simulink model "Target_Control_System"  (R2021b)
settings: Solver=FixedStepDiscrete  StartTime=0.0  StopTime=5  RelTol=1e-3
PreLoadFcn:
  | RTWConfigurationCB('preloadfcn', bdroot);
PostLoadFcn:
  | load('configuration/data_struct.mat');
  | load('configuration/fluxMaps_propMotor.mat');
  | load('configuration/parameterInit_PROP.mat');
  | load('configuration/parameterInit_PUMP.mat');
  | load('configuration/parameterInit_PITCH.mat');
  | load('configuration/parameterInit_TILT.mat');
  | %load('configuration/base_workspace_signal_definition.mat');
  | %load('resolvedatastores_to_baseworkspace_for_faster_simulation.mat');
model workspace (MAT data in the model file):
  SIMULATION_OPTIONS : Simulink.Parameter (value not decoded)
  TARGET_CODE_GEN : Simulink.Parameter (value not decoded)
  TCS_SAMPLE_FREQ_HZ : Simulink.Parameter (value not decoded)
symbols that are objects in the model workspace (value not decoded): TARGET_CODE_GEN, TCS_SAMPLE_FREQ_HZ
undefined symbols (not defined in the file): A_DQ_REF_LPF_INIT__PITCH, A_DQ_REF_LPF_INIT__PROP, A_DQ_REF_LPF_INIT__PUMP, A_DQ_REF_LPF_INIT__TILT, A_OBSERVER_CONFIDENCE_INIT__PITCH, A_OBSERVER_CONFIDENCE_INIT__PROP, A_OBSERVER_CONFIDENCE_INIT__PUMP, A_OBSERVER_CONFIDENCE_INIT__TILT, ACTUATOR_MAX_ANGLE_TRIP__PITCH, ACTUATOR_MIN_ANGLE_TRIP__PITCH, ACTUATOR_POS_SENSOR_INV_DIRECTION__PITCH, ACTUATOR_POS_SENSOR_INV_DIRECTION__TILT, ACTUATOR_POS_SENSOR_OFFSET__PITCH, ACTUATOR_POS_SENSOR_OFFSET__TILT, ADC_scaler1_baseaddr_TILT, ADC_SCALER_FLOAT_TO_FIXPOINT_EXPANSION, ANGLE_ELEC_FROM_SENSOR_OFFSET_INIT__PITCH, ANGLE_ELEC_FROM_SENSOR_OFFSET_INIT__PROP, ANGLE_ELEC_FROM_SENSOR_OFFSET_INIT__PUMP, ANGLE_ELEC_FROM_SENSOR_OFFSET_INIT__TILT, AUTO_CLEAR_FAULTS_ENABLED__PITCH, AUTO_CLEAR_FAULTS_ENABLED__PROP, AUTO_CLEAR_FAULTS_ENABLED__PUMP, AUTO_CLEAR_FAULTS_ENABLED__TILT, AUTO_CLEAR_FAULTS_WAIT_TICKS__PITCH, AUTO_CLEAR_FAULTS_WAIT_TICKS__PROP, AUTO_CLEAR_FAULTS_WAIT_TICKS__PUMP, AUTO_CLEAR_FAULTS_WAIT_TICKS__TILT, AUTO_I_ZERO_IDLE_TICKS__PITCH, AUTO_I_ZERO_IDLE_TICKS__PROP, AUTO_I_ZERO_IDLE_TICKS__PUMP, AUTO_I_ZERO_IDLE_TICKS__TILT, AUTO_I_ZERO_OFFSET_IDC_THRESHOLD__PITCH, AUTO_I_ZERO_OFFSET_IDC_THRESHOLD__PROP, AUTO_I_ZERO_OFFSET_IDC_THRESHOLD__PUMP, AUTO_I_ZERO_OFFSET_IDC_THRESHOLD__TILT, AUTO_I_ZERO_OFFSET_IPH_THRESHOLD__PITCH, AUTO_I_ZERO_OFFSET_IPH_THRESHOLD__PROP, AUTO_I_ZERO_OFFSET_IPH_THRESHOLD__PUMP, AUTO_I_ZERO_OFFSET_IPH_THRESHOLD__TILT, AUTO_SENSORLESS_SWITCHOVER_DISABLE_OMEGA, AUTO_SENSORLESS_SWITCHOVER_ENABLE_OMEGA, AUTO_SENSORLESS_SWITCHOVER_MIN_CONFIDENCE, AUXILIARY_PROTECTION_UNIT_BASEADDR__TILT, blanking_max_error_omega_INIT_PITCH, blanking_max_error_omega_INIT_TILT, blanking_max_error_position_INIT_PITCH, blanking_max_error_position_INIT_TILT, BRUTE_START_I_Q_REF_RAMP_SPEED__PITCH, BRUTE_START_I_Q_REF_RAMP_SPEED__PROP, BRUTE_START_I_Q_REF_RAMP_SPEED__PUMP, BRUTE_START_I_Q_REF_RAMP_SPEED__TILT, CONTROL_LOOP_DT_INIT__PITCH, CONTROL_LOOP_DT_INIT__PROP, CONTROL_LOOP_DT_INIT__PUMP, CONTROL_LOOP_DT_INIT__TILT, CORRECTION_FILTER_SCALE__PITCH, CORRECTION_FILTER_SCALE__PROP, CORRECTION_FILTER_SCALE__PUMP, CORRECTION_FILTER_SCALE__TILT ... (+458)
libraries: simulink x178, Reusables_Lib x24
(part 7 of 47)

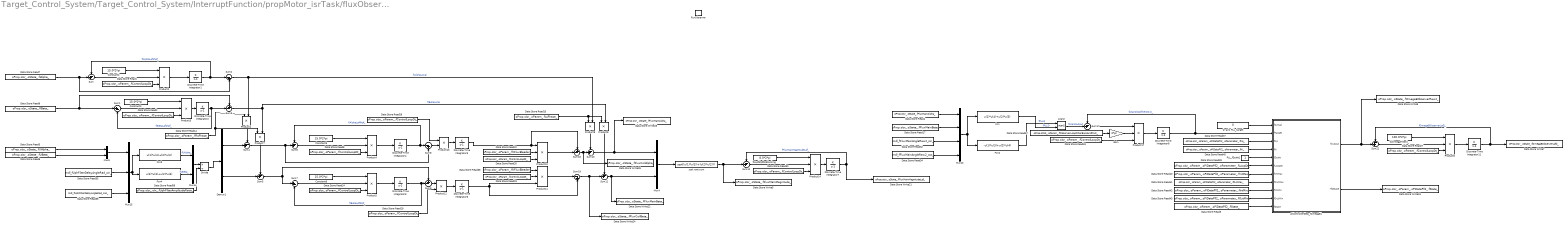
== system Target_Control_System/Target_Control_System/InterruptFunction/propMotor_isrTask/fluxObserver ==
  fluxObserver : TriggerPort  TriggerType=function-call  VariantControl=Variant
  Atan2 : Trigonometry  Operator=atan2
  Constant{2..3,5..6} (4 alike) : Constant  Value=15.0*2*pi  OutDataTypeStr=single  SampleTime=-1
  Data Store Read{1..2,8,20,23..24,27..30,33} (11 alike) : DataStoreRead  DataStoreName=oProp  DataStoreElements=oProp.oIsr_.oParam_.fControlLoopDt_  IndexOptions=Index vector (dialog)  Indices=1  OutputSizes=1
  Data Store Read14 : DataStoreRead  DataStoreName=oProp  DataStoreElements=oProp.oIsr_.oParam_.fRsPhase_  IndexOptions=Index vector (dialog)  Indices=1  OutputSizes=1
  Data Store Read15 : DataStoreRead  DataStoreName=oProp  DataStoreElements=oProp.oIsr_.oParam_.fLsPhase_  IndexOptions=Index vector (dialog)  Indices=1  OutputSizes=1
  Data Store Read17 : DataStoreRead  DataStoreName=oProp  DataStoreElements=oProp.oIsr_.oState_.fFluxMainBeta_  IndexOptions=Index vector (dialog)  Indices=1  OutputSizes=1
  Data Store Read22 : DataStoreRead  DataStoreName=oProp  DataStoreElements=oProp.oIsr_.oParam_.fKFluxBleeder_  IndexOptions=Index vector (dialog)  Indices=1  OutputSizes=1
  Data Store Read3 : DataStoreRead  DataStoreName=oProp  DataStoreElements=oProp.oIsr_.oParam_.oPiDataPll2_.fState_  IndexOptions=Index vector (dialog)  Indices=1  OutputSizes=1
  Data Store Read32 : DataStoreRead  DataStoreName=mdl_fFluxMainAngleRaw2_sin_  IndexOptions=Index vector (dialog)  Indices=1  OutputSizes=1
  Data Store Read34 : DataStoreRead  DataStoreName=mdl_fFluxMainAngleRaw2_cos_  IndexOptions=Index vector (dialog)  Indices=1  OutputSizes=1
  Data Store Read35 : DataStoreRead  DataStoreName=mdl_fUphFilterDelayAngleRad_sin_  IndexOptions=Index vector (dialog)  Indices=1  OutputSizes=1
  Data Store Read36 : DataStoreRead  DataStoreName=mdl_fUphFilterDelayAngleRad_cos_  IndexOptions=Index vector (dialog)  Indices=1  OutputSizes=1
  Data Store Read37 : DataStoreRead  DataStoreName=oProp  DataStoreElements=oProp.oIsr_.oParam_.oPiDataPll2_.oParameter_.fKp_  IndexOptions=Index vector (dialog)  Indices=1  OutputSizes=1
  Data Store Read38 : DataStoreRead  DataStoreName=oProp  DataStoreElements=oProp.oIsr_.oParam_.fKFluxBleeder_  IndexOptions=Index vector (dialog)  Indices=1  OutputSizes=1
  Data Store Read39 : DataStoreRead  DataStoreName=oProp  DataStoreElements=oProp.oIsr_.oParam_.oPiDataPll2_.oParameter_.fLoopDt_  IndexOptions=Index vector (dialog)  Indices=1  OutputSizes=1
  Data Store Read4 : DataStoreRead  DataStoreName=oProp  DataStoreElements=oProp.oIsr_.oState_.fFluxMainAlpha_  IndexOptions=Index vector (dialog)  Indices=1  OutputSizes=1
  Data Store Read40 : DataStoreRead  DataStoreName=oProp  DataStoreElements=oProp.oIsr_.oParam_.oPiDataPll2_.oParameter_.fIntMax_  IndexOptions=Index vector (dialog)  Indices=1  OutputSizes=1
  Data Store Read41 : DataStoreRead  DataStoreName=oProp  DataStoreElements=oProp.oIsr_.oParam_.oPiDataPll2_.oParameter_.fOutMax_  IndexOptions=Index vector (dialog)  Indices=1  OutputSizes=1
  Data Store Read42 : DataStoreRead  DataStoreName=oProp  DataStoreElements=oProp.oIsr_.oParam_.oPiDataPll2_.oParameter_.fIntMin_  IndexOptions=Index vector (dialog)  Indices=1  OutputSizes=1
  Data Store Read43 : DataStoreRead  DataStoreName=oProp  DataStoreElements=oProp.oIsr_.oParam_.oPiDataPll2_.oParameter_.fOutMin_  IndexOptions=Index vector (dialog)  Indices=1  OutputSizes=1
  Data Store Read45 : DataStoreRead  DataStoreName=oProp  DataStoreElements=oProp.oIsr_.oParam_.oPiDataPll2_.oParameter_.fKi_  IndexOptions=Index vector (dialog)  Indices=1  OutputSizes=1
  Data Store Read5 : DataStoreRead  DataStoreName=oProp  DataStoreElements=oProp.oIsr_.oState_.fUAlpha_  IndexOptions=Index vector (dialog)  Indices=1  OutputSizes=1
  Data Store Read57 : DataStoreRead  DataStoreName=oProp  DataStoreElements=oProp.oMot_.oParam_.fObserverLoopFilterBandwidthHz_  IndexOptions=Index vector (dialog)  Indices=1  OutputSizes=1
  Data Store Read58 : DataStoreRead  DataStoreName=oProp  DataStoreElements=oProp.oIsr_.oIn_.fUphFilterAmplitudeRatio_  IndexOptions=Index vector (dialog)  Indices=1  OutputSizes=1
  Data Store Read6 : DataStoreRead  DataStoreName=oProp  DataStoreElements=oProp.oIsr_.oState_.fUBeta_  IndexOptions=Index vector (dialog)  Indices=1  OutputSizes=1
  Data Store Read7 : DataStoreRead  DataStoreName=oProp  DataStoreElements=oProp.oIsr_.oState_.fIAlpha_  IndexOptions=Index vector (dialog)  Indices=1  OutputSizes=1
  Data Store Read9 : DataStoreRead  DataStoreName=oProp  DataStoreElements=oProp.oIsr_.oState_.fIBeta_  IndexOptions=Index vector (dialog)  Indices=1  OutputSizes=1
  Data Store Write19 : DataStoreWrite  DataStoreName=oProp  DataStoreElements=oProp.oIsr_.oParam_.oPiDataPll2_.fState_  IndexOptions=Index vector (dialog)  Indices=1  OutputSizes=1
  Data Store Write21 : DataStoreWrite  DataStoreName=oProp  DataStoreElements=oProp.oIsr_.oState_.fFluxMainMagnitudeLpf_  IndexOptions=Index vector (dialog)  Indices=1  OutputSizes=1
  Data Store Write22 : DataStoreWrite  DataStoreName=oProp  DataStoreElements=oProp.oIsr_.oState_.fFluxMainBeta_  IndexOptions=Index vector (dialog)  Indices=1  OutputSizes=1
  Data Store Write23 : DataStoreWrite  DataStoreName=oProp  DataStoreElements=oProp.oIsr_.oState_.fFluxMainAlpha_  IndexOptions=Index vector (dialog)  Indices=1  OutputSizes=1
  Data Store Write24 : DataStoreWrite  DataStoreName=oProp  DataStoreElements=oProp.oIsr_.oState_.fFluxCoilBeta_  IndexOptions=Index vector (dialog)  Indices=1  OutputSizes=1
  Data Store Write26 : DataStoreWrite  DataStoreName=oProp  DataStoreElements=oProp.oIsr_.oState_.fFluxCoilAlpha_  IndexOptions=Index vector (dialog)  Indices=1  OutputSizes=1
  Data Store Write5 : DataStoreWrite  DataStoreName=oProp  DataStoreElements=oProp.oIsr_.oState_.fFluxMainMagnitude_  IndexOptions=Index vector (dialog)  Indices=1  OutputSizes=1
  Data Store Write7 : DataStoreWrite  DataStoreName=oProp  DataStoreElements=oProp.oIsr_.oState_.fOmegaEObserverLpf2_  IndexOptions=Index vector (dialog)  Indices=1  OutputSizes=1
  Data Store Write9 : DataStoreWrite  DataStoreName=oProp  DataStoreElements=oProp.oIsr_.oState_.fOmegaEObserverRaw2_  IndexOptions=Index vector (dialog)  Indices=1  OutputSizes=1
  Demux1 : Demux  Outputs=2
  Discrete-Time Integrator{1..2,4..9,11} (9 alike) : DiscreteIntegrator  IntegratorMethod=Accumulation: Forward Euler  SampleTime=-1  OutDataTypeStr=single  UpperSaturationLimit=2*pi*100  LowerSaturationLimit=-2*pi*100  ICPrevOutput=DiscIntNeverNeededParam  ICPrevScaledInput=DiscIntNeverNeededParam
  Divide : Product  Inputs=*/
  Fcn : Fcn  Expr=u(1)*u(4)+u(2)*u(3)
  Fcn2 : Fcn  Expr=-u(1)*u(3)+u(2)*u(4)
  Fcn3 : Fcn  Expr=u(1)*u(4)-u(2)*u(3)
  Fcn4 : Fcn  Expr=u(1)*u(3)+u(2)*u(4)
  Gain : Gain  Gain=2*pi
  Mux13 : Mux
  Mux14 : Mux  Inputs=2
  Mux15 : Mux  Inputs=3
  Mux4 : Mux  Inputs=2
  Mux5 : Mux  Inputs=2
  PLL_fScale1 : Constant  OutDataTypeStr=single  SampleTime=-1
  Product{1,7..9,12..13} (6 alike) : Product
  Product{2..6,10..11,14,17} (9 alike) : Product  Inputs=3
  Q-axis PLL_target : Constant  Value=0  OutDataTypeStr=single  SampleTime=-1
  Sum{,4..6,10..12,17,22} (9 alike) : Sum  Inputs=-+|
  Sum1 : Sum  Inputs=|+-
  Sum18 : Sum  Inputs=+-|
  Sum19 : Sum  Inputs=|-+
  Sum2 : Sum  Inputs=|-+
  Sum3 : Sum  Inputs=+-|
  Sum7 : Sum  Inputs=|+-
  Sum8 : Sum  Inputs=|-+
  Sum9 : Sum  Inputs=+-|
  fALpf4hpfDcBlocking : Constant  Value=8.0*2*pi  OutDataTypeStr=single  SampleTime=-1
  fAOmegaFilter2_ : Constant  Value=100.0*2*pi  OutDataTypeStr=single  SampleTime=-1
  piControllerStep_fOmegaE1 : Subsystem
  sqrt root sum : Fcn  Expr=sqrt((u(1)*u(1))+(u(2)*u(2)))
  wires:
  Data Store Read29/1 -> Product12/2
  Data Store Read35/1 -> Mux15/2
  Data Store Read24/1 -> Product5/3
  Constant5/1 -> Product4/1
  Mux15/1 -> Fcn4/1, Fcn3/1
  Product7/1 -> Sum5/1
  Data Store Read57/1 -> Gain/1
  Mux4/1 -> sqrt root sum/1
  Discrete-Time Integrator2/1 -> Sum1/2, Sum3/2  "fIBetaLpf4hpf_"
  Constant6/1 -> Product5/1
  Sum3/1 -> Product9/2, Product7/2  "fIBetaLocal"
  Sum7/1 -> Product5/2
  Sum2/1 -> Product1/2, Product8/2  "fIAlphaLocal"
  Data Store Read5/1 -> Mux5/1
  Product11/1 -> Sum19/1
  Sum6/1 -> Product4/2
  Discrete-Time Integrator1/1 -> Sum2/1, Sum/1  "fIAlphaLpf4hpf_"
  fALpf4hpfDcBlocking/1 -> Product14/1
  Sum10/1 -> Mux4/1, Data Store Write23/1
  Data Store Read28/1 -> Product13/1
  Sum1/1 -> Product3/2
  Data Store Read1/1 -> Product2/3
  Data Store Read43/1 -> piControllerStep_fOmegaE1/10(fOutMin)
  Demux1/1 -> Sum4/2
  Data Store Read38/1 -> Product11/1
  Discrete-Time Integrator6/1 -> Sum19/2, Product11/3
  Divide/1 -> Demux1/1
  Product13/1 -> Discrete-Time Integrator5/1
  Data Store Read36/1 -> Mux15/3
  Mux14/1 -> Divide/1
  Data Store Read40/1 -> piControllerStep_fOmegaE1/7(fIntMax)
  Data Store Read45/1 -> piControllerStep_fOmegaE1/4(fKi)
  fAOmegaFilter2_/1 -> Product6/1
  Data Store Read17/1 -> Mux13/2
  Product1/1 -> Sum4/1
  Data Store Read39/1 -> piControllerStep_fOmegaE1/6(fLoopDt)
  Data Store Read7/1 -> Sum2/2, Sum/2
  Sum19/1 -> Sum11/2, Data Store Write24/1
  Sum18/1 -> Sum10/2, Data Store Write26/1
  Data Store Read34/1 -> Mux13/4
  Product17/1 -> Discrete-Time Integrator8/1
  piControllerStep_fOmegaE1/1(fOutput) -> Sum22/2, Data Store Write9/1
  Data Store Read8/1 -> Product4/3
  Atan2/1 -> Sum17/2  "fAtan2output"
  Product2/1 -> Discrete-Time Integrator1/1
  Data Store Read14/1 -> Product1/1, Product7/1
  Fcn4/1 -> Mux14/2  "fUBeta_"
  Data Store Read20/1 -> Product10/3
  Discrete-Time Integrator5/1 -> Sum18/1, Product10/1
  Demux1/2 -> Sum5/2
  Product10/1 -> Sum18/2
  Sum17/1 -> Product17/1
  Product8/1 -> Sum10/1
  Discrete-Time Integrator11/1 -> Sum22/1, Data Store Write7/1  "fOmegaEObserverLpf2_"
  Mux13/1 -> Fcn2/1, Fcn/1
  Q-axis PLL_target/1 -> piControllerStep_fOmegaE1/1(fActual)
  Fcn3/1 -> Mux14/1  "fUAlpha_"
  Data Store Read42/1 -> piControllerStep_fOmegaE1/9(fIntMin)
  Sum4/1 -> Sum8/2, Sum6/2
  Constant3/1 -> Product3/1
  Fcn/1 -> Atan2/2  "fPLLD"
  Product6/1 -> Discrete-Time Integrator11/1
  Data Store Read2/1 -> Product3/3
  Discrete-Time Integrator9/1 -> Sum9/2, Sum7/2  "fIBetaLpf4hpf_"
  Sum5/1 -> Sum9/1, Sum7/1
  Mux5/1 -> Mux15/1
  Data Store Read58/1 -> Divide/2
  Sum12/1 -> Product14/2
  Sum22/1 -> Product6/2
  Fcn2/1 -> Atan2/1  "fPLLQ"
  sqrt root sum/1 -> Data Store Write5/1, Sum12/2
  Data Store Read23/1 -> Product11/2
  PLL_fScale1/1 -> piControllerStep_fOmegaE1/5(fScale)
  Data Store Read22/1 -> Product10/2
  Product12/1 -> Discrete-Time Integrator6/1
  Discrete-Time Integrator8/1 -> piControllerStep_fOmegaE1/2(fTarget), Sum17/1  "fAtan2loopfilter2Out_"
  Sum/1 -> Product2/2
  Sum9/1 -> Product12/1
  Data Store Read3/1 -> piControllerStep_fOmegaE1/11(fState)
  Gain/1 -> Product17/2
  Sum8/1 -> Product13/2
  Sum11/1 -> Mux4/2, Data Store Write22/1
  Data Store Read15/1 -> Product8/1, Product9/1
  Product5/1 -> Discrete-Time Integrator9/1
  Discrete-Time Integrator4/1 -> Sum8/1, Sum6/1  "fIAlphaLpf4hpf_"
  Constant2/1 -> Product2/1
  Discrete-Time Integrator7/1 -> Data Store Write21/1, Sum12/1  "fFluxMainMagnitudeLpf_"
  Data Store Read6/1 -> Mux5/2
  Data Store Read32/1 -> Mux13/3
  Data Store Read27/1 -> Product6/3
  Product4/1 -> Discrete-Time Integrator4/1
  Data Store Read4/1 -> Mux13/1
  Data Store Read33/1 -> Product17/3
  Data Store Read30/1 -> Product14/3
  piControllerStep_fOmegaE1/2(*fpState) -> Data Store Write19/1
  Data Store Read37/1 -> piControllerStep_fOmegaE1/3(fKp)
  Product9/1 -> Sum11/1
  Product3/1 -> Discrete-Time Integrator2/1
  Product14/1 -> Discrete-Time Integrator7/1
  Data Store Read41/1 -> piControllerStep_fOmegaE1/8(fOutMax)
  Data Store Read9/1 -> Sum1/1, Sum3/1

== system Target_Control_System/Target_Control_System/InterruptFunction/propMotor_isrTask/isrStateMachine ==
  isrStateMachine : TriggerPort  TriggerType=function-call  VariantControl=Variant
  ISR State Machine : Stateflow chart  TreatAsAtomicUnit=on

== system Target_Control_System/Target_Control_System/InterruptFunction/propMotor_isrTask/pwmGeneration ==
  pwmGeneration : TriggerPort  TriggerType=function-call  VariantControl=Variant
  Data Store Read9 : DataStoreRead  DataStoreName=oProp  DataStoreElements=oProp.oIsr_.oIn_.uiCurrentControllerActive_  IndexOptions=Index vector (dialog)  Indices=1  OutputSizes=1
  Subsystem : Subsystem
  wires:
  Data Store Read9/1 -> Subsystem/Enable

== system Target_Control_System/Target_Control_System/InterruptFunction/propMotor_isrTask/resetFlags ==
  resetFlags : TriggerPort  TriggerType=function-call  VariantControl=Variant
  Constant : Constant  Value=0  OutDataTypeStr=int32  SampleTime=-1
  Data Store Write1 : DataStoreWrite  DataStoreName=oProp  DataStoreElements=oProp.oIsr_.oOut_.iIBiasUpdated_  IndexOptions=Index vector (dialog)  Indices=1  OutputSizes=1
  Data Store Write12 : DataStoreWrite  DataStoreName=oProp  DataStoreElements=oProp.oIsr_.oState_.iPwmUpdated_  IndexOptions=Index vector (dialog)  Indices=1  OutputSizes=1
  Data Store Write2 : DataStoreWrite  DataStoreName=oProp  DataStoreElements=oProp.oIsr_.oOut_.iUBiasUpdated_  IndexOptions=Index vector (dialog)  Indices=1  OutputSizes=1
  wires:
  Constant/1 -> Data Store Write12/1, Data Store Write1/1, Data Store Write2/1

== system Target_Control_System/Target_Control_System/InterruptFunction/propMotor_isrTask/softCurrentLimiting ==
  softCurrentLimiting : TriggerPort  TriggerType=function-call  VariantControl=Variant
  Abs : Abs
  Abs1 : Abs
  Abs2 : Abs
  Add : Sum  Inputs=+-
  Add1 : Sum  Inputs=+-
  Add2 : Sum  Inputs=+-
  Constant : Constant  Value=0  OutDataTypeStr=single  SampleTime=-1
  Data Store Read1 : DataStoreRead  DataStoreName=oProp  DataStoreElements=oProp.oIsr_.oIn_.oAdcData_.fIa_  IndexOptions=Index vector (dialog)  Indices=1  OutputSizes=1
  Data Store Read2 : DataStoreRead  DataStoreName=oProp  DataStoreElements=oProp.oIsr_.oParam_.fSoftILimitA_  IndexOptions=Index vector (dialog)  Indices=1  OutputSizes=1
  Data Store Read3 : DataStoreRead  DataStoreName=oProp  DataStoreElements=oProp.oIsr_.oIn_.oAdcData_.fIb_  IndexOptions=Index vector (dialog)  Indices=1  OutputSizes=1
  Data Store Read4 : DataStoreRead  DataStoreName=oProp  DataStoreElements=oProp.oIsr_.oParam_.fSoftILimitA_  IndexOptions=Index vector (dialog)  Indices=1  OutputSizes=1
  Data Store Read5 : DataStoreRead  DataStoreName=oProp  DataStoreElements=oProp.oIsr_.oIn_.oAdcData_.fIc_  IndexOptions=Index vector (dialog)  Indices=1  OutputSizes=1
  Data Store Read6 : DataStoreRead  DataStoreName=oProp  DataStoreElements=oProp.oIsr_.oParam_.fSoftILimitA_  IndexOptions=Index vector (dialog)  Indices=1  OutputSizes=1
  Equal : RelationalOperator  Operator=>  OutDataTypeStr=boolean  RndMeth=Simplest
  Equal1 : RelationalOperator  Operator=>  OutDataTypeStr=boolean  RndMeth=Simplest
  Equal2 : RelationalOperator  Operator=>  OutDataTypeStr=boolean  RndMeth=Simplest
  Subsystem : Subsystem
  Switch : Switch  Criteria=u2 > Threshold
  Switch1 : Switch  Criteria=u2 > Threshold
  wires:
  Equal/1 -> Switch/2
  Data Store Read6/1 -> Add2/2
  Data Store Read5/1 -> Abs2/1
  Equal1/1 -> Switch1/2
  Abs1/1 -> Add1/1
  Add/1 -> Equal/2, Switch/3  "fMaxOvershoot"
  Constant/1 -> Equal2/2
  Abs/1 -> Add/1
  Add2/1 -> Switch1/1, Equal1/1  "fTemp"
  Switch1/1 -> Equal2/1, Subsystem/1(fMaxOvershoot)  "fMaxOvershoot"
  Data Store Read3/1 -> Abs1/1
  Add1/1 -> Switch/1, Equal/1  "fTemp"
  Switch/1 -> Switch1/3, Equal1/2  "fMaxOvershoot"
  Equal2/1 -> Subsystem/Enable
  Data Store Read1/1 -> Abs/1
  Abs2/1 -> Add2/1
  Data Store Read4/1 -> Add1/2
  Data Store Read2/1 -> Add/2

== system Target_Control_System/Target_Control_System/InterruptFunction/propMotor_setPwm/ModelSourceFPGAProp ==
  note: 1) Add Subsystem or Model blocks as valid variant choices.
      | 2) You cannot connect blocks at this level. At simulation, connectivity is automatically
      | determined, based on the active variant and port name matching.
  DoNotIncludeCustomCode : Subsystem  TreatAsAtomicUnit=on  VariantControl=TARGET_CODE_GEN == 0
  IncludeCustomCode : Subsystem  TreatAsAtomicUnit=on  VariantControl=(default)

== system Target_Control_System/Target_Control_System/InterruptFunction/propMotor_setPwm/Subsystem ==
  note: // signal to the pwm block that we handled the interrupt
  Enable : EnablePort
  Constant10 : Constant  OutDataTypeStr=int32  SampleTime=-1
  Data Store Read2 : DataStoreRead  DataStoreName=oProp  DataStoreElements=oProp.oIsr_.oParam_.fPwmPeriodTicksFloat_  IndexOptions=Index vector (dialog)  Indices=1  OutputSizes=1
  Data Store Write : DataStoreWrite  DataStoreName=oProp  DataStoreElements=oProp.oIsr_.oOut_.uiPwmDutyTicksA_  IndexOptions=Index vector (dialog)  Indices=1  OutputSizes=1
  Data Type Conversion : DataTypeConversion  OutDataTypeStr=uint32
  Shift Arithmetic1 : ArithShift  BitShiftNumberSource=Input port  BitShiftNumber=8  BitShiftDirection=Right
      settings: InputPortMap=u0,p1
  wires:
  Shift Arithmetic1/1 -> Data Type Conversion/1
  Data Type Conversion/1 -> Data Store Write/1
  Data Store Read2/1 -> Shift Arithmetic1/1
  Constant10/1 -> Shift Arithmetic1/2

== system Target_Control_System/Target_Control_System/InterruptFunction/pumpMotor_isrSchedule/Triggered Subsystem ==
  Trigger : TriggerPort  VariantControl=Variant
  Function-Call Generator : simulink/Ports & Subsystems/Function-Call Generator  sample_time=-1  numberOfIterations=1  DisallowWideOutput=off
  Output : Outport
  wires:
  Function-Call Generator/1 -> Output/1

== system Target_Control_System/Target_Control_System/InterruptFunction/pumpMotor_isrTask/abcToAlphaBeta ==
  abcToAlphaBeta : TriggerPort  TriggerType=function-call  VariantControl=Variant
  Constant1 : Constant  Value=TARGET_CODE_GEN  SampleTime=-1
  Data Store Read1 : DataStoreRead  DataStoreName=oPump  DataStoreElements=oPump.oIsr_.oState_.fUaPostlpf_  IndexOptions=Index vector (dialog)  Indices=1  OutputSizes=1
  Data Store Read13 : DataStoreRead  DataStoreName=oPump  DataStoreElements=oPump.oIsr_.oState_.fUbPostlpf_  IndexOptions=Index vector (dialog)  Indices=1  OutputSizes=1
  Data Store Read14 : DataStoreRead  DataStoreName=oPump  DataStoreElements=oPump.oIsr_.oState_.fUcPostlpf_  IndexOptions=Index vector (dialog)  Indices=1  OutputSizes=1
  Data Store Read15 : DataStoreRead  DataStoreName=oPump  DataStoreElements=oPump.oIsr_.oIn_.fUphFilterDelayAngleRad_  IndexOptions=Index vector (dialog)  Indices=1  OutputSizes=1
  Data Store Read16 : DataStoreRead  DataStoreName=oPump  DataStoreElements=oPump.oIsr_.oIn_.oAdcData_.fIa_  IndexOptions=Index vector (dialog)  Indices=1  OutputSizes=1
  Data Store Read17 : DataStoreRead  DataStoreName=oPump  DataStoreElements=oPump.oIsr_.oState_.fOmegaEObserverRaw2_  IndexOptions=Index vector (dialog)  Indices=1  OutputSizes=1
  Data Store Read19 : DataStoreRead  DataStoreName=oPump  DataStoreElements=oPump.oIsr_.oParam_.iInverseDirection_  IndexOptions=Index vector (dialog)  Indices=1  OutputSizes=1
  Data Store Read2 : DataStoreRead  DataStoreName=oPump  DataStoreElements=oPump.oIsr_.oIn_.oAdcData_.fIb_  IndexOptions=Index vector (dialog)  Indices=1  OutputSizes=1
  Data Store Read4 : DataStoreRead  DataStoreName=oPump  DataStoreElements=oPump.oIsr_.oIn_.oAdcData_.fIc_  IndexOptions=Index vector (dialog)  Indices=1  OutputSizes=1
  Data Store Read8 : DataStoreRead  DataStoreName=oPump  DataStoreElements=oPump.oIsr_.oParam_.iInverseDirection_  IndexOptions=Index vector (dialog)  Indices=1  OutputSizes=1
  Data Store Write1 : DataStoreWrite  DataStoreName=oPump  DataStoreElements=oPump.oIsr_.oState_.fIAlpha_  IndexOptions=Index vector (dialog)  Indices=1  OutputSizes=1
  Data Store Write2 : DataStoreWrite  DataStoreName=oPump  DataStoreElements=oPump.oIsr_.oState_.fFluxMainAngleRaw2_  IndexOptions=Index vector (dialog)  Indices=1  OutputSizes=1
  Data Store Write3 : DataStoreWrite  DataStoreName=oPump  DataStoreElements=oPump.oIsr_.oState_.fIBeta_  IndexOptions=Index vector (dialog)  Indices=1  OutputSizes=1
  Data Store Write4 : DataStoreWrite  DataStoreName=oPump  DataStoreElements=oPump.oIsr_.oState_.fUBeta_  IndexOptions=Index vector (dialog)  Indices=1  OutputSizes=1
  Data Store Write5 : DataStoreWrite  DataStoreName=oPump  DataStoreElements=oPump.oIsr_.oState_.fUAlpha_  IndexOptions=Index vector (dialog)  Indices=1  OutputSizes=1
  Demux3 : Demux  Outputs=2
  Demux4 : Demux  Outputs=2
  Integrator with Angle Wrapper : Subsystem
  Integrator with Angle Wrapper_OLD : Subsystem  Commented=on
  ModelSource : Subsystem  Variant=on
  Mux2 : Mux  Inputs=3
  Mux4 : Mux  Inputs=3
  NOT1 : Logic  Operator=NOT  AllPortsSameDT=off  OutDataTypeStr=boolean
  Switch2 : Switch  Criteria=u2 > Threshold
  Switch3 : Switch  Criteria=u2 > Threshold
  abc to alpha/beta2 : Gain  Gain="2/3*[1 -0.5 -0.5  ; 0 sqrt(3)/2 -sqrt(3)/2 ]"  Multiplication=Matrix(K*u) (u vector)
  abc to alpha/beta3 : Gain  Gain="2/3*[1 -0.5 -0.5  ; 0 sqrt(3)/2 -sqrt(3)/2 ]"  Multiplication=Matrix(K*u) (u vector)
  abc to alpha/beta_inverseDirection2 : Gain  Gain="2/3*[1 -0.5 -0.5  ; 0 -sqrt(3)/2 sqrt(3)/2 ]"  Multiplication=Matrix(K*u) (u vector)
  abc to alpha/beta_inverseDirection3 : Gain  Gain="2/3*[1 -0.5 -0.5  ; 0 -sqrt(3)/2 sqrt(3)/2 ]"  Multiplication=Matrix(K*u) (u vector)
  vsincos()1 : Subsystem  TreatAsAtomicUnit=on
  wires:
  Data Store Read14/1 -> Mux4/3
  Data Store Read1/1 -> Mux4/1
  abc to alpha/beta3/1 -> Switch2/3
  Data Store Read2/1 -> Mux2/2
  Data Store Read19/1 -> Switch2/2
  Mux2/1 -> abc to alpha/beta3/1, abc to alpha/beta_inverseDirection2/1
  Demux3/1 -> Data Store Write1/1
  Switch2/1 -> Demux3/1
  abc to alpha/beta_inverseDirection3/1 -> Switch3/1
  NOT1/1 -> vsincos()1/Enable
  Constant1/1 -> NOT1/1
  Demux3/2 -> Data Store Write3/1
  Integrator with Angle Wrapper/1(Angle) -> vsincos()1/2(Input1), Data Store Write2/1  "fFluxMainAngleRaw2_"
  Data Store Read17/1 -> Integrator with Angle Wrapper/1(Omega)
  abc to alpha/beta2/1 -> Switch3/3
  Switch3/1 -> Demux4/1
  Data Store Read16/1 -> Mux2/1
  Data Store Read15/1 -> vsincos()1/1(Input)
  Data Store Read8/1 -> Switch3/2
  abc to alpha/beta_inverseDirection2/1 -> Switch2/1
  Data Store Read4/1 -> Mux2/3
  Mux4/1 -> abc to alpha/beta_inverseDirection3/1, abc to alpha/beta2/1
  Data Store Read13/1 -> Mux4/2
  Demux4/2 -> Data Store Write4/1
  Demux4/1 -> Data Store Write5/1

== system Target_Control_System/Target_Control_System/InterruptFunction/pumpMotor_isrTask/currentController ==
  currentController : TriggerPort  TriggerType=function-call  VariantControl=Variant
  Data Store Read9 : DataStoreRead  DataStoreName=oPump  DataStoreElements=oPump.oIsr_.oIn_.uiCurrentControllerActive_  IndexOptions=Index vector (dialog)  Indices=1  OutputSizes=1
  Subsystem : Subsystem
  wires:
  Data Store Read9/1 -> Subsystem/Enable

== system Target_Control_System/Target_Control_System/InterruptFunction/pumpMotor_isrTask/dqTransform ==
  dqTransform : TriggerPort  TriggerType=function-call  VariantControl=Variant
  Data Store Read13 : DataStoreRead  DataStoreName=mdl_pump_fFluxMasterAngle_cos_  IndexOptions=Index vector (dialog)  Indices=1  OutputSizes=1
  Data Store Read16 : DataStoreRead  DataStoreName=oPump  DataStoreElements=oPump.oIsr_.oState_.fIAlpha_  IndexOptions=Index vector (dialog)  Indices=1  OutputSizes=1
  Data Store Read24 : DataStoreRead  DataStoreName=oPump  DataStoreElements=oPump.oIsr_.oState_.fIq_  IndexOptions=Index vector (dialog)  Indices=1  OutputSizes=1
  Data Store Read3 : DataStoreRead  DataStoreName=mdl_pump_fFluxMasterAngle_sin_  IndexOptions=Index vector (dialog)  Indices=1  OutputSizes=1
  Data Store Read30 : DataStoreRead  DataStoreName=oPump  DataStoreElements=oPump.oIsr_.oState_.fFluxMainMagnitudeLpf_  IndexOptions=Index vector (dialog)  Indices=1  OutputSizes=1
  Data Store Read32 : DataStoreRead  DataStoreName=oPump  DataStoreElements=oPump.oIsr_.oState_.fIBeta_  IndexOptions=Index vector (dialog)  Indices=1  OutputSizes=1
  Data Store Read61 : DataStoreRead  DataStoreName=oPump  DataStoreElements=oPump.oIsr_.oParam_.fPolePairs_  IndexOptions=Index vector (dialog)  Indices=1  OutputSizes=1
  Data Store Write1 : DataStoreWrite  DataStoreName=oPump  DataStoreElements=oPump.oIsr_.oState_.fId_  IndexOptions=Index vector (dialog)  Indices=1  OutputSizes=1
  Data Store Write10 : DataStoreWrite  DataStoreName=oPump  DataStoreElements=oPump.oIsr_.oOut_.fIPhaseMagnitude_  IndexOptions=Index vector (dialog)  Indices=1  OutputSizes=1
  Data Store Write33 : DataStoreWrite  DataStoreName=oPump  DataStoreElements=oPump.oIsr_.oOut_.fTEstimate_  IndexOptions=Index vector (dialog)  Indices=1  OutputSizes=1
  Data Store Write9 : DataStoreWrite  DataStoreName=oPump  DataStoreElements=oPump.oIsr_.oState_.fIq_  IndexOptions=Index vector (dialog)  Indices=1  OutputSizes=1
  Fcn5 : Fcn  Expr=3/2*u(1)*u(2)*u(3)
  Mux2 : Mux  Inputs=2
  Mux5 : Mux
  Mux6 : Mux  Inputs=3
  Square Root Sum : Fcn  Expr=sqrt((u(1)*u(1))+(u(2)*u(2)))
  fId_ = fCosTerm*opState->fIAlpha_ + fSinTerm*opState->fIBeta_1 : Fcn  Expr=u(4)*u(1)+u(3)*u(2)
  fIq_ = fCosTerm*opState->fIBeta_ - fSinTerm*opState->fIAlpha_1 : Fcn  Expr=u(4)*u(2)-u(3)*u(1)
  wires:
  fId_ = fCosTerm*opState->fIAlpha_ + fSinTerm*opState->fIBeta_1/1 -> Mux2/1, Data Store Write1/1
  Data Store Read13/1 -> Mux5/4
  Data Store Read3/1 -> Mux5/3
  Data Store Read24/1 -> Mux6/3
  Data Store Read16/1 -> Mux5/1
  Data Store Read32/1 -> Mux5/2
  Data Store Read30/1 -> Mux6/2
  Mux2/1 -> Square Root Sum/1
  Mux6/1 -> Fcn5/1
  Fcn5/1 -> Data Store Write33/1
  Data Store Read61/1 -> Mux6/1
  Square Root Sum/1 -> Data Store Write10/1
  Mux5/1 -> fId_ = fCosTerm*opState->fIAlpha_ + fSinTerm*opState->fIBeta_1/1, fIq_ = fCosTerm*opState->fIBeta_ - fSinTerm*opState->fIAlpha_1/1
  fIq_ = fCosTerm*opState->fIBeta_ - fSinTerm*opState->fIAlpha_1/1 -> Mux2/2, Data Store Write9/1

== system Target_Control_System/Target_Control_System/InterruptFunction/pumpMotor_isrTask/fluxAngleCalculations ==
  fluxAngleCalculation : TriggerPort  TriggerType=function-call  VariantControl=Variant
  Add1 : Sum
  Angle Clip1 : Subsystem
  Constant5 : Constant  Value=TARGET_CODE_GEN  SampleTime=-1
  Data Store Read2 : DataStoreRead  DataStoreName=oPump  DataStoreElements=oPump.oIsr_.oState_.fFluxMainAngleRaw2_  IndexOptions=Index vector (dialog)  Indices=1  OutputSizes=1
  Data Store Read3 : DataStoreRead  DataStoreName=oPump  DataStoreElements=oPump.oIsr_.oState_.fOmegaEObserverLpf2_  IndexOptions=Index vector (dialog)  Indices=1  OutputSizes=1
  Data Store Read4 : DataStoreRead  DataStoreName=oPump  DataStoreElements=oPump.oIsr_.oIn_.uiForcedAngle_  IndexOptions=Index vector (dialog)  Indices=1  OutputSizes=1
  Data Store Read5 : DataStoreRead  DataStoreName=oPump  DataStoreElements=oPump.oIsr_.oIn_.fOmegaERefRampOut_  IndexOptions=Index vector (dialog)  Indices=1  OutputSizes=1
  Data Store Read6 : DataStoreRead  DataStoreName=oPump  DataStoreElements=oPump.oIsr_.oIn_.fFluxMasterAngleOffsetRampOut_  IndexOptions=Index vector (dialog)  Indices=1  OutputSizes=1
  Data Store Read7 : DataStoreRead  DataStoreName=oPump  DataStoreElements=oPump.oIsr_.oIn_.fFluxMasterAngleForced2closedSmoothingRampOut_  IndexOptions=Index vector (dialog)  Indices=1  OutputSizes=1
  Data Store Write3 : DataStoreWrite  DataStoreName=oPump  DataStoreElements=oPump.oIsr_.oState_.fFluxMasterAngle_  IndexOptions=Index vector (dialog)  Indices=1  OutputSizes=1
  Data Store Write4 : DataStoreWrite  DataStoreName=oPump  DataStoreElements=oPump.oIsr_.oState_.fFluxMasterAngleBkwd_  IndexOptions=Index vector (dialog)  Indices=1  OutputSizes=1
  Data Store Write5 : DataStoreWrite  DataStoreName=mdl_pump_fOmegaE  IndexOptions=Index vector (dialog)  Indices=1  OutputSizes=1
  Equal1 : RelationalOperator  Operator===  OutDataTypeStr=boolean  RndMeth=Simplest
  Equal3 : RelationalOperator  Operator=~=  OutDataTypeStr=boolean  RndMeth=Simplest
  ModelSource1 : Subsystem  Variant=on
  NOT2 : Logic  Operator=NOT  AllPortsSameDT=off  OutDataTypeStr=boolean
  One1 : Constant  OutDataTypeStr=uint32  SampleTime=-1
  Subsystem2 : Subsystem
  Subsystem3 : Subsystem
  Switch1 : Switch  Criteria=u2 > Threshold  Threshold=0.5
  Switch2 : Switch  Criteria=u2 > Threshold  Threshold=0.5
  Switch3 : Switch  Criteria=u2 > Threshold  Threshold=0.5
  Zero2 : Constant  Value=0  OutDataTypeStr=single  SampleTime=-1
  vsincos()2 : Subsystem  TreatAsAtomicUnit=on
  wires:
  Data Store Read3/1 -> Switch3/3
  Add1/1 -> Angle Clip1/1(Angle_In)
  Switch1/1 -> Switch2/3, Subsystem3/1(In1)
  Data Store Read6/1 -> Add1/2
  Angle Clip1/1(Angle_Out) -> vsincos()2/2(fFluxMasterAngleBdwd), Data Store Write4/1
  One1/1 -> Equal1/2
  Data Store Read2/1 -> Switch1/3  "fFluxMainAngleRaw2_"
  Equal1/1 -> Switch1/2, Switch3/2, Subsystem2/Enable
  Subsystem3/1(Angle_Out) -> Switch2/1
  Constant5/1 -> NOT2/1
  Data Store Read7/1 -> Subsystem3/2(In2), Equal3/1
  Data Store Read5/1 -> Switch3/1
  Equal3/1 -> Switch2/2, Subsystem3/Enable
  Switch2/1 -> vsincos()2/1(fFluxMasterAngle), Data Store Write3/1, Add1/1
  Data Store Read4/1 -> Equal1/1
  Switch3/1 -> Data Store Write5/1  "fFluxMasterAngle_"
  NOT2/1 -> vsincos()2/Enable
  Zero2/1 -> Equal3/2
  Subsystem2/1(Angle) -> Switch1/1

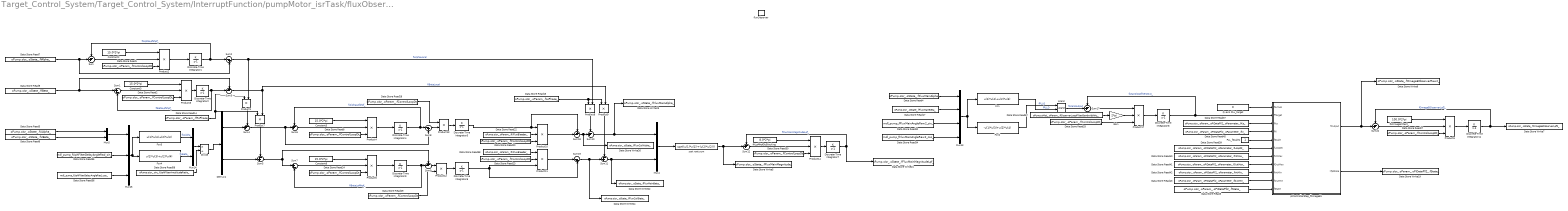
== system Target_Control_System/Target_Control_System/InterruptFunction/pumpMotor_isrTask/fluxObserver ==
  fluxObserver : TriggerPort  TriggerType=function-call  VariantControl=Variant
  Atan2 : Trigonometry  Operator=atan2
  Constant{2..3,5..6} (4 alike) : Constant  Value=15.0*2*pi  OutDataTypeStr=single  SampleTime=-1
  Data Store Read{1..2,8,20,23..24,27..30,33} (11 alike) : DataStoreRead  DataStoreName=oPump  DataStoreElements=oPump.oIsr_.oParam_.fControlLoopDt_  IndexOptions=Index vector (dialog)  Indices=1  OutputSizes=1
  Data Store Read14 : DataStoreRead  DataStoreName=oPump  DataStoreElements=oPump.oIsr_.oParam_.fRsPhase_  IndexOptions=Index vector (dialog)  Indices=1  OutputSizes=1
  Data Store Read15 : DataStoreRead  DataStoreName=oPump  DataStoreElements=oPump.oIsr_.oParam_.fLsPhase_  IndexOptions=Index vector (dialog)  Indices=1  OutputSizes=1
  Data Store Read17 : DataStoreRead  DataStoreName=oPump  DataStoreElements=oPump.oIsr_.oState_.fFluxMainBeta_  IndexOptions=Index vector (dialog)  Indices=1  OutputSizes=1
  Data Store Read22 : DataStoreRead  DataStoreName=oPump  DataStoreElements=oPump.oIsr_.oParam_.fKFluxBleeder_  IndexOptions=Index vector (dialog)  Indices=1  OutputSizes=1
  Data Store Read3 : DataStoreRead  DataStoreName=oPump  DataStoreElements=oPump.oIsr_.oParam_.oPiDataPll2_.fState_  IndexOptions=Index vector (dialog)  Indices=1  OutputSizes=1
  Data Store Read32 : DataStoreRead  DataStoreName=mdl_pump_fFluxMainAngleRaw2_sin_  IndexOptions=Index vector (dialog)  Indices=1  OutputSizes=1
  Data Store Read34 : DataStoreRead  DataStoreName=mdl_pump_fFluxMainAngleRaw2_cos_  IndexOptions=Index vector (dialog)  Indices=1  OutputSizes=1
  Data Store Read35 : DataStoreRead  DataStoreName=mdl_pump_fUphFilterDelayAngleRad_sin_  IndexOptions=Index vector (dialog)  Indices=1  OutputSizes=1
  Data Store Read36 : DataStoreRead  DataStoreName=mdl_pump_fUphFilterDelayAngleRad_cos_  IndexOptions=Index vector (dialog)  Indices=1  OutputSizes=1
  Data Store Read37 : DataStoreRead  DataStoreName=oPump  DataStoreElements=oPump.oIsr_.oParam_.oPiDataPll2_.oParameter_.fKp_  IndexOptions=Index vector (dialog)  Indices=1  OutputSizes=1
  Data Store Read38 : DataStoreRead  DataStoreName=oPump  DataStoreElements=oPump.oIsr_.oParam_.fKFluxBleeder_  IndexOptions=Index vector (dialog)  Indices=1  OutputSizes=1
  Data Store Read39 : DataStoreRead  DataStoreName=oPump  DataStoreElements=oPump.oIsr_.oParam_.oPiDataPll2_.oParameter_.fLoopDt_  IndexOptions=Index vector (dialog)  Indices=1  OutputSizes=1
  Data Store Read4 : DataStoreRead  DataStoreName=oPump  DataStoreElements=oPump.oIsr_.oState_.fFluxMainAlpha_  IndexOptions=Index vector (dialog)  Indices=1  OutputSizes=1
  Data Store Read40 : DataStoreRead  DataStoreName=oPump  DataStoreElements=oPump.oIsr_.oParam_.oPiDataPll2_.oParameter_.fIntMax_  IndexOptions=Index vector (dialog)  Indices=1  OutputSizes=1
  Data Store Read41 : DataStoreRead  DataStoreName=oPump  DataStoreElements=oPump.oIsr_.oParam_.oPiDataPll2_.oParameter_.fOutMax_  IndexOptions=Index vector (dialog)  Indices=1  OutputSizes=1
  Data Store Read42 : DataStoreRead  DataStoreName=oPump  DataStoreElements=oPump.oIsr_.oParam_.oPiDataPll2_.oParameter_.fIntMin_  IndexOptions=Index vector (dialog)  Indices=1  OutputSizes=1
  Data Store Read43 : DataStoreRead  DataStoreName=oPump  DataStoreElements=oPump.oIsr_.oParam_.oPiDataPll2_.oParameter_.fOutMin_  IndexOptions=Index vector (dialog)  Indices=1  OutputSizes=1
  Data Store Read45 : DataStoreRead  DataStoreName=oPump  DataStoreElements=oPump.oIsr_.oParam_.oPiDataPll2_.oParameter_.fKi_  IndexOptions=Index vector (dialog)  Indices=1  OutputSizes=1
  Data Store Read5 : DataStoreRead  DataStoreName=oPump  DataStoreElements=oPump.oIsr_.oState_.fUAlpha_  IndexOptions=Index vector (dialog)  Indices=1  OutputSizes=1
  Data Store Read57 : DataStoreRead  DataStoreName=oPump  DataStoreElements=oPump.oMot_.oParam_.fObserverLoopFilterBandwidthHz_  IndexOptions=Index vector (dialog)  Indices=1  OutputSizes=1
  Data Store Read58 : DataStoreRead  DataStoreName=oPump  DataStoreElements=oPump.oIsr_.oIn_.fUphFilterAmplitudeRatio_  IndexOptions=Index vector (dialog)  Indices=1  OutputSizes=1
  Data Store Read6 : DataStoreRead  DataStoreName=oPump  DataStoreElements=oPump.oIsr_.oState_.fUBeta_  IndexOptions=Index vector (dialog)  Indices=1  OutputSizes=1
  Data Store Read7 : DataStoreRead  DataStoreName=oPump  DataStoreElements=oPump.oIsr_.oState_.fIAlpha_  IndexOptions=Index vector (dialog)  Indices=1  OutputSizes=1
  Data Store Read9 : DataStoreRead  DataStoreName=oPump  DataStoreElements=oPump.oIsr_.oState_.fIBeta_  IndexOptions=Index vector (dialog)  Indices=1  OutputSizes=1
  Data Store Write19 : DataStoreWrite  DataStoreName=oPump  DataStoreElements=oPump.oIsr_.oParam_.oPiDataPll2_.fState_  IndexOptions=Index vector (dialog)  Indices=1  OutputSizes=1
  Data Store Write21 : DataStoreWrite  DataStoreName=oPump  DataStoreElements=oPump.oIsr_.oState_.fFluxMainMagnitudeLpf_  IndexOptions=Index vector (dialog)  Indices=1  OutputSizes=1
  Data Store Write22 : DataStoreWrite  DataStoreName=oPump  DataStoreElements=oPump.oIsr_.oState_.fFluxMainBeta_  IndexOptions=Index vector (dialog)  Indices=1  OutputSizes=1
  Data Store Write23 : DataStoreWrite  DataStoreName=oPump  DataStoreElements=oPump.oIsr_.oState_.fFluxMainAlpha_  IndexOptions=Index vector (dialog)  Indices=1  OutputSizes=1
  Data Store Write24 : DataStoreWrite  DataStoreName=oPump  DataStoreElements=oPump.oIsr_.oState_.fFluxCoilBeta_  IndexOptions=Index vector (dialog)  Indices=1  OutputSizes=1
  Data Store Write26 : DataStoreWrite  DataStoreName=oPump  DataStoreElements=oPump.oIsr_.oState_.fFluxCoilAlpha_  IndexOptions=Index vector (dialog)  Indices=1  OutputSizes=1
  Data Store Write5 : DataStoreWrite  DataStoreName=oPump  DataStoreElements=oPump.oIsr_.oState_.fFluxMainMagnitude_  IndexOptions=Index vector (dialog)  Indices=1  OutputSizes=1
  Data Store Write7 : DataStoreWrite  DataStoreName=oPump  DataStoreElements=oPump.oIsr_.oState_.fOmegaEObserverLpf2_  IndexOptions=Index vector (dialog)  Indices=1  OutputSizes=1
  Data Store Write9 : DataStoreWrite  DataStoreName=oPump  DataStoreElements=oPump.oIsr_.oState_.fOmegaEObserverRaw2_  IndexOptions=Index vector (dialog)  Indices=1  OutputSizes=1
  Demux1 : Demux  Outputs=2
  Discrete-Time Integrator{1..2,4..9,11} (9 alike) : DiscreteIntegrator  IntegratorMethod=Accumulation: Forward Euler  SampleTime=-1  OutDataTypeStr=single  UpperSaturationLimit=2*pi*100  LowerSaturationLimit=-2*pi*100  ICPrevOutput=DiscIntNeverNeededParam  ICPrevScaledInput=DiscIntNeverNeededParam
  Divide : Product  Inputs=*/
  Fcn : Fcn  Expr=u(1)*u(4)+u(2)*u(3)
  Fcn2 : Fcn  Expr=-u(1)*u(3)+u(2)*u(4)
  Fcn3 : Fcn  Expr=u(1)*u(4)-u(2)*u(3)
  Fcn4 : Fcn  Expr=u(1)*u(3)+u(2)*u(4)
  Gain : Gain  Gain=2*pi
  Mux13 : Mux
  Mux14 : Mux  Inputs=2
  Mux15 : Mux  Inputs=3
  Mux4 : Mux  Inputs=2
  Mux5 : Mux  Inputs=2
  PLL_fScale1 : Constant  OutDataTypeStr=single  SampleTime=-1
  Product{1,7..9,12..13} (6 alike) : Product
  Product{2..6,10..11,14,17} (9 alike) : Product  Inputs=3
  Q-axis PLL_target : Constant  Value=0  OutDataTypeStr=single  SampleTime=-1
  Sum{,4..6,10..12,17,22} (9 alike) : Sum  Inputs=-+|
  Sum1 : Sum  Inputs=|+-
  Sum18 : Sum  Inputs=+-|
  Sum19 : Sum  Inputs=|-+
  Sum2 : Sum  Inputs=|-+
  Sum3 : Sum  Inputs=+-|
  Sum7 : Sum  Inputs=|+-
  Sum8 : Sum  Inputs=|-+
  Sum9 : Sum  Inputs=+-|
  fALpf4hpfDcBlocking : Constant  Value=8.0*2*pi  OutDataTypeStr=single  SampleTime=-1
  fAOmegaFilter2_ : Constant  Value=100.0*2*pi  OutDataTypeStr=single  SampleTime=-1
  piControllerStep_fOmegaE1 : Subsystem
  sqrt root sum : Fcn  Expr=sqrt((u(1)*u(1))+(u(2)*u(2)))
  wires:
  Mux5/1 -> Mux15/1
  Discrete-Time Integrator8/1 -> piControllerStep_fOmegaE1/2(fTarget), Sum17/1  "fAtan2loopfilter2Out_"
  PLL_fScale1/1 -> piControllerStep_fOmegaE1/5(fScale)
  Data Store Read45/1 -> piControllerStep_fOmegaE1/4(fKi)
  Data Store Read17/1 -> Mux13/2
  Data Store Read40/1 -> piControllerStep_fOmegaE1/7(fIntMax)
  Sum6/1 -> Product4/2
  Product1/1 -> Sum4/1
  Gain/1 -> Product17/2
  Discrete-Time Integrator4/1 -> Sum8/1, Sum6/1  "fIAlphaLpf4hpf_"
  Product17/1 -> Discrete-Time Integrator8/1
  Sum3/1 -> Product9/2, Product7/2  "fIBetaLocal"
  Mux15/1 -> Fcn4/1, Fcn3/1
  Sum5/1 -> Sum9/1, Sum7/1
  Sum11/1 -> Mux4/2, Data Store Write22/1
  Data Store Read14/1 -> Product1/1, Product7/1
  Data Store Read30/1 -> Product14/3
  Discrete-Time Integrator1/1 -> Sum2/1, Sum/1  "fIAlphaLpf4hpf_"
  Data Store Read43/1 -> piControllerStep_fOmegaE1/10(fOutMin)
  Q-axis PLL_target/1 -> piControllerStep_fOmegaE1/1(fActual)
  Data Store Read28/1 -> Product13/1
  Data Store Read23/1 -> Product11/2
  Data Store Read42/1 -> piControllerStep_fOmegaE1/9(fIntMin)
  Sum8/1 -> Product13/2
  Sum12/1 -> Product14/2
  Data Store Read32/1 -> Mux13/3
  Data Store Read15/1 -> Product8/1, Product9/1
  Discrete-Time Integrator6/1 -> Sum19/2, Product11/3
  Sum1/1 -> Product3/2
  Fcn4/1 -> Mux14/2  "fUBeta_"
  Mux13/1 -> Fcn2/1, Fcn/1
  Data Store Read24/1 -> Product5/3
  Sum7/1 -> Product5/2
  Sum4/1 -> Sum8/2, Sum6/2
  Data Store Read37/1 -> piControllerStep_fOmegaE1/3(fKp)
  Constant2/1 -> Product2/1
  Constant3/1 -> Product3/1
  Data Store Read5/1 -> Mux5/1
  Product13/1 -> Discrete-Time Integrator5/1
  Constant5/1 -> Product4/1
  Data Store Read29/1 -> Product12/2
  Data Store Read2/1 -> Product3/3
  Discrete-Time Integrator9/1 -> Sum9/2, Sum7/2  "fIBetaLpf4hpf_"
  Product9/1 -> Sum11/1
  Fcn/1 -> Atan2/2  "fPLLD"
  Product12/1 -> Discrete-Time Integrator6/1
  Data Store Read36/1 -> Mux15/3
  Product7/1 -> Sum5/1
  Data Store Read7/1 -> Sum2/2, Sum/2
  Data Store Read6/1 -> Mux5/2
  Data Store Read57/1 -> Gain/1
  Product3/1 -> Discrete-Time Integrator2/1
  Sum18/1 -> Sum10/2, Data Store Write26/1
  Sum22/1 -> Product6/2
  Discrete-Time Integrator5/1 -> Sum18/1, Product10/1
  Data Store Read27/1 -> Product6/3
  Product10/1 -> Sum18/2
  Mux14/1 -> Divide/1
  Data Store Read35/1 -> Mux15/2
  Data Store Read1/1 -> Product2/3
  Discrete-Time Integrator2/1 -> Sum1/2, Sum3/2  "fIBetaLpf4hpf_"
  Data Store Read3/1 -> piControllerStep_fOmegaE1/11(fState)
  piControllerStep_fOmegaE1/1(fOutput) -> Sum22/2, Data Store Write9/1
  Constant6/1 -> Product5/1
  Discrete-Time Integrator11/1 -> Sum22/1, Data Store Write7/1  "fOmegaEObserverLpf2_"
  Product8/1 -> Sum10/1
  Sum19/1 -> Sum11/2, Data Store Write24/1
  Data Store Read58/1 -> Divide/2
  Demux1/1 -> Sum4/2
  Data Store Read22/1 -> Product10/2
  Product6/1 -> Discrete-Time Integrator11/1
  Fcn2/1 -> Atan2/1  "fPLLQ"
  fAOmegaFilter2_/1 -> Product6/1
  fALpf4hpfDcBlocking/1 -> Product14/1
  Data Store Read38/1 -> Product11/1
  Data Store Read8/1 -> Product4/3
  Product5/1 -> Discrete-Time Integrator9/1
  Sum/1 -> Product2/2
  Sum17/1 -> Product17/1
  Product11/1 -> Sum19/1
  Data Store Read41/1 -> piControllerStep_fOmegaE1/8(fOutMax)
  Product14/1 -> Discrete-Time Integrator7/1
  sqrt root sum/1 -> Data Store Write5/1, Sum12/2
  Data Store Read34/1 -> Mux13/4
  Divide/1 -> Demux1/1
  Data Store Read4/1 -> Mux13/1
  Sum10/1 -> Mux4/1, Data Store Write23/1
  Sum9/1 -> Product12/1
  Data Store Read9/1 -> Sum1/1, Sum3/1
  Product4/1 -> Discrete-Time Integrator4/1
  Data Store Read39/1 -> piControllerStep_fOmegaE1/6(fLoopDt)
  Mux4/1 -> sqrt root sum/1
  piControllerStep_fOmegaE1/2(*fpState) -> Data Store Write19/1
  Demux1/2 -> Sum5/2
  Sum2/1 -> Product1/2, Product8/2  "fIAlphaLocal"
  Product2/1 -> Discrete-Time Integrator1/1
  Data Store Read33/1 -> Product17/3
  Discrete-Time Integrator7/1 -> Data Store Write21/1, Sum12/1  "fFluxMainMagnitudeLpf_"
  Fcn3/1 -> Mux14/1  "fUAlpha_"
  Atan2/1 -> Sum17/2  "fAtan2output"
  Data Store Read20/1 -> Product10/3

== system Target_Control_System/Target_Control_System/InterruptFunction/pumpMotor_isrTask/isrStateMachine ==
  isrStateMachine : TriggerPort  TriggerType=function-call  VariantControl=Variant
  ISR State Machine : Stateflow chart  TreatAsAtomicUnit=on

== system Target_Control_System/Target_Control_System/InterruptFunction/pumpMotor_isrTask/pwmGeneration ==
  pwmGeneration : TriggerPort  TriggerType=function-call  VariantControl=Variant
  Data Store Read9 : DataStoreRead  DataStoreName=oPump  DataStoreElements=oPump.oIsr_.oIn_.uiCurrentControllerActive_  IndexOptions=Index vector (dialog)  Indices=1  OutputSizes=1
  Subsystem : Subsystem
  wires:
  Data Store Read9/1 -> Subsystem/Enable

== system Target_Control_System/Target_Control_System/InterruptFunction/pumpMotor_isrTask/resetFlags ==
  resetFlags : TriggerPort  TriggerType=function-call  VariantControl=Variant
  Constant : Constant  Value=0  OutDataTypeStr=int32  SampleTime=-1
  Data Store Write1 : DataStoreWrite  DataStoreName=oPump  DataStoreElements=oPump.oIsr_.oOut_.iIBiasUpdated_  IndexOptions=Index vector (dialog)  Indices=1  OutputSizes=1
  Data Store Write12 : DataStoreWrite  DataStoreName=oPump  DataStoreElements=oPump.oIsr_.oState_.iPwmUpdated_  IndexOptions=Index vector (dialog)  Indices=1  OutputSizes=1
  Data Store Write2 : DataStoreWrite  DataStoreName=oPump  DataStoreElements=oPump.oIsr_.oOut_.iUBiasUpdated_  IndexOptions=Index vector (dialog)  Indices=1  OutputSizes=1
  wires:
  Constant/1 -> Data Store Write12/1, Data Store Write1/1, Data Store Write2/1

== system Target_Control_System/Target_Control_System/InterruptFunction/pumpMotor_isrTask/softCurrentLimiting ==
  softCurrentLimiting : TriggerPort  TriggerType=function-call  VariantControl=Variant
  Abs : Abs
  Abs1 : Abs
  Abs2 : Abs
  Add : Sum  Inputs=+-
  Add1 : Sum  Inputs=+-
  Add2 : Sum  Inputs=+-
  Constant : Constant  Value=0  OutDataTypeStr=single  SampleTime=-1
  Data Store Read1 : DataStoreRead  DataStoreName=oPump  DataStoreElements=oPump.oIsr_.oIn_.oAdcData_.fIa_  IndexOptions=Index vector (dialog)  Indices=1  OutputSizes=1
  Data Store Read2 : DataStoreRead  DataStoreName=oPump  DataStoreElements=oPump.oIsr_.oParam_.fSoftILimitA_  IndexOptions=Index vector (dialog)  Indices=1  OutputSizes=1
  Data Store Read3 : DataStoreRead  DataStoreName=oPump  DataStoreElements=oPump.oIsr_.oIn_.oAdcData_.fIb_  IndexOptions=Index vector (dialog)  Indices=1  OutputSizes=1
  Data Store Read4 : DataStoreRead  DataStoreName=oPump  DataStoreElements=oPump.oIsr_.oParam_.fSoftILimitA_  IndexOptions=Index vector (dialog)  Indices=1  OutputSizes=1
  Data Store Read5 : DataStoreRead  DataStoreName=oPump  DataStoreElements=oPump.oIsr_.oIn_.oAdcData_.fIc_  IndexOptions=Index vector (dialog)  Indices=1  OutputSizes=1
  Data Store Read6 : DataStoreRead  DataStoreName=oPump  DataStoreElements=oPump.oIsr_.oParam_.fSoftILimitA_  IndexOptions=Index vector (dialog)  Indices=1  OutputSizes=1
  Equal : RelationalOperator  Operator=>  OutDataTypeStr=boolean  RndMeth=Simplest
  Equal1 : RelationalOperator  Operator=>  OutDataTypeStr=boolean  RndMeth=Simplest
  Equal2 : RelationalOperator  Operator=>  OutDataTypeStr=boolean  RndMeth=Simplest
  Subsystem : Subsystem
  Switch : Switch  Criteria=u2 > Threshold
  Switch1 : Switch  Criteria=u2 > Threshold
  wires:
  Constant/1 -> Equal2/2
  Switch/1 -> Switch1/3, Equal1/2  "fMaxOvershoot"
  Data Store Read3/1 -> Abs1/1
  Data Store Read2/1 -> Add/2
  Add1/1 -> Switch/1, Equal/1  "fTemp"
  Equal2/1 -> Subsystem/Enable
  Data Store Read4/1 -> Add1/2
  Add/1 -> Equal/2, Switch/3  "fMaxOvershoot"
  Equal1/1 -> Switch1/2
  Abs1/1 -> Add1/1
  Switch1/1 -> Equal2/1, Subsystem/1(fMaxOvershoot)  "fMaxOvershoot"
  Data Store Read6/1 -> Add2/2
  Data Store Read1/1 -> Abs/1
  Data Store Read5/1 -> Abs2/1
  Equal/1 -> Switch/2
  Add2/1 -> Switch1/1, Equal1/1  "fTemp"
  Abs2/1 -> Add2/1
  Abs/1 -> Add/1

== system Target_Control_System/Target_Control_System/InterruptFunction/pumpMotor_setPwm/ModelSourceFPGAPump ==
  note: 1) Add Subsystem or Model blocks as valid variant choices.
      | 2) You cannot connect blocks at this level. At simulation, connectivity is automatically
      | determined, based on the active variant and port name matching.
  DoNotIncludeCustomCode : Subsystem  TreatAsAtomicUnit=on  VariantControl=TARGET_CODE_GEN == 0
  IncludeCustomCode : Subsystem  TreatAsAtomicUnit=on  VariantControl=(default)

== system Target_Control_System/Target_Control_System/InterruptFunction/pumpMotor_setPwm/Subsystem ==
  note: // signal to the pwm block that we handled the interrupt
  Enable : EnablePort
  Constant10 : Constant  OutDataTypeStr=int32  SampleTime=-1
  Data Store Read2 : DataStoreRead  DataStoreName=oPump  DataStoreElements=oPump.oIsr_.oParam_.fPwmPeriodTicksFloat_  IndexOptions=Index vector (dialog)  Indices=1  OutputSizes=1
  Data Store Write : DataStoreWrite  DataStoreName=oPump  DataStoreElements=oPump.oIsr_.oOut_.uiPwmDutyTicksA_  IndexOptions=Index vector (dialog)  Indices=1  OutputSizes=1
  Data Type Conversion : DataTypeConversion  OutDataTypeStr=uint32
  Shift Arithmetic1 : ArithShift  BitShiftNumberSource=Input port  BitShiftNumber=8  BitShiftDirection=Right
      settings: InputPortMap=u0,p1
  wires:
  Shift Arithmetic1/1 -> Data Type Conversion/1
  Data Type Conversion/1 -> Data Store Write/1
  Data Store Read2/1 -> Shift Arithmetic1/1
  Constant10/1 -> Shift Arithmetic1/2
